simulink model "BuckyWagon_01"  (Simulink 7.5)
settings: Solver=FixedStepDiscrete  StartTime=0.0  StopTime=10.0  RelTol=1e-3
PreLoadFcn:
  | try, eval([bdroot '_setup']); catch, eval('model_setup', ''); end
InitFcn:
  | try, eval([bdroot '_setup']); catch, eval('model_setup', ''); end
undefined symbols (not defined in the file): ECU565, High, Low, miniviewSetup, motohawk_build_version, motohawk_get_faults, motohawk_setup_toolchains, motohawk_trunc_name, motohawk_vardec_config_group, motohawk_vardec_path, tc, True
libraries: MotoHawk_lib x499, simulink x29, motohawk_engine_lib x19, miniview_lib x10, motohawk_control_primitives_lib x8, motohawk_annotations_lib x2
(part 8 of 9)

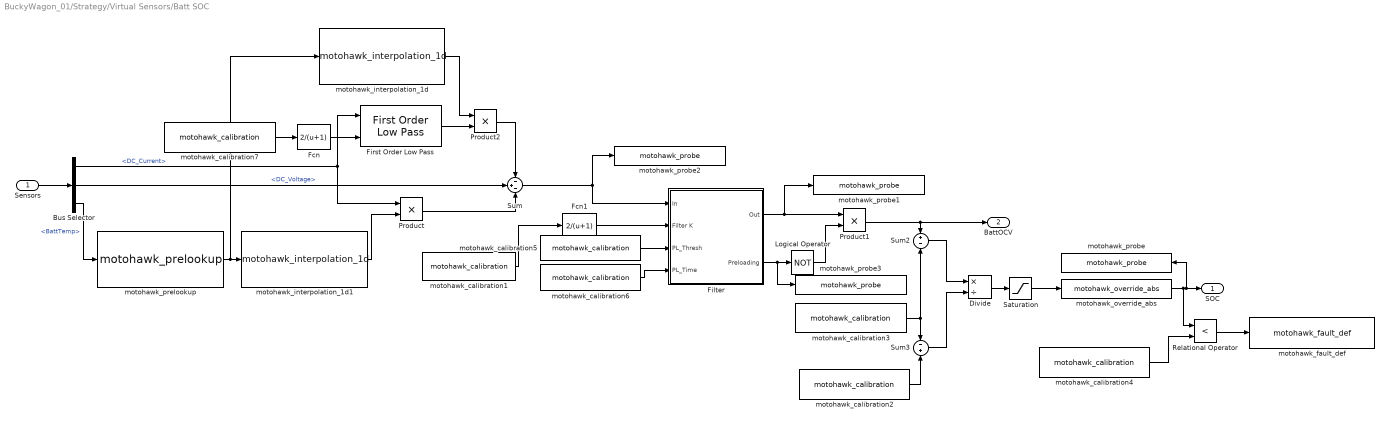
== system BuckyWagon_01/Strategy/Virtual Sensors/Batt SOC ==
  Sensors : Inport  OutDataType=sfix(16)  OutScaling=2^0
  Bus Selector : BusSelector  OutputSignals=DC_Current,DC_Voltage,BattTemp
  Divide : Product  Inputs=*/  OutDataType=sfix(16)  OutScaling=2^-10
  Fcn : Fcn  Expr=2/(u+1)
  Fcn1 : Fcn  Expr=2/(u+1)
  Filter : Subsystem
  First Order Low Pass : motohawk_control_primitives_lib/First Order Low Pass  SystemSampleTime=-1
  Logical Operator : Logic  Operator=NOT  AllPortsSameDT=off  OutDataTypeMode=boolean  OutDataTypeStr=boolean
  Product : Product  OutDataType=sfix(16)  OutScaling=2^0  RndMeth=Zero
  Product1 : Product  OutDataType=sfix(16)  OutScaling=2^0  RndMeth=Zero
  Product2 : Product  OutDataType=sfix(16)  OutScaling=2^0  RndMeth=Zero
  Relational Operator : RelationalOperator  Operator=<  LogicOutDataTypeMode=boolean  OutDataTypeStr=boolean
  Saturation : Saturate  UpperLimit=1  LowerLimit=0  OutDataType=sfix(16)  OutScaling=2^0
  Sum : Sum  Inputs=-+-  OutDataType=sfix(16)  OutScaling=2^0
  Sum2 : Sum  Inputs=+-  OutDataType=sfix(16)  OutScaling=2^0
  Sum3 : Sum  Inputs=-+  OutDataType=sfix(16)  OutScaling=2^0
  motohawk_calibration1 : MotoHawk_lib/Calibration & Probing Blocks/motohawk_calibration  nam='BattV_TC'  val=10/0.005  storage=Calibration  show_more=on  name_source=Use Parameter  data_type=Inherit from 'Default Value'  read_level=1  write_level=1  ovr_cals=on  view_as=Number  enum_struct={'Disabled', 'Enabled'}  vector_style=Wide Row  use_help_units=on  help='Filter on Batt OCV Time Constant.'  units='s'  use_header_enum=off  row_header_enum={}  col_header_enum={}  use_min_max=on  min_val=0.005  max_val=inf  use_precision=on  precision='1.5'  gain=0.005  offset=0  exp=1  use_mototune_group=off  mototune_group=motohawk_vardec_path(gcb)
  motohawk_calibration2 : MotoHawk_lib/Calibration & Probing Blocks/motohawk_calibration  nam='Batt_Full_V'  val=350  storage=Calibration  show_more=on  name_source=Use Parameter  data_type=Inherit from 'Default Value'  read_level=1  write_level=1  ovr_cals=on  view_as=Number  enum_struct={'Disabled', 'Enabled'}  vector_style=Wide Row  use_help_units=on  help='100% SOC Voltage'  units='V'  use_header_enum=off  row_header_enum={}  col_header_enum={}  use_min_max=off  min_val=-inf  max_val=inf  use_precision=on  precision='3.1'  gain=1  offset=0  exp=1  use_mototune_group=off  mototune_group=motohawk_vardec_path(gcb)
  motohawk_calibration3 : MotoHawk_lib/Calibration & Probing Blocks/motohawk_calibration  nam='Batt_Empty_V'  val=350  storage=Calibration  show_more=on  name_source=Use Parameter  data_type=Inherit from 'Default Value'  read_level=1  write_level=1  ovr_cals=on  view_as=Number  enum_struct={'Disabled', 'Enabled'}  vector_style=Wide Row  use_help_units=on  help='0% SOC Voltage'  units='V'  use_header_enum=off  row_header_enum={}  col_header_enum={}  use_min_max=off  min_val=-inf  max_val=inf  use_precision=on  precision='3.1'  gain=1  offset=0  exp=1  use_mototune_group=off  mototune_group=motohawk_vardec_path(gcb)
  motohawk_calibration4 : MotoHawk_lib/Calibration & Probing Blocks/motohawk_calibration  nam='SOC_Dead'  val=0.1  storage=Calibration  show_more=on  name_source=Use Parameter  data_type=Inherit from 'Default Value'  read_level=1  write_level=1  ovr_cals=on  view_as=Number  enum_struct={'Disabled', 'Enabled'}  vector_style=Wide Row  use_help_units=on  help='Below this SOC a Batt Dead fault will occur.'  units='%'  use_header_enum=off  row_header_enum={}  col_header_enum={}  use_min_max=on  min_val=0  max_val=1  use_precision=on  precision='1.3'  gain=1  offset=0  exp=1  use_mototune_group=off  mototune_group=motohawk_vardec_path(gcb)
  motohawk_calibration5 : MotoHawk_lib/Calibration & Probing Blocks/motohawk_calibration  nam='BattVFilt_PreLThres'  val=100  storage=Calibration  show_more=on  name_source=Use Parameter  data_type=Inherit from 'Default Value'  read_level=1  write_level=1  ovr_cals=on  view_as=Number  enum_struct={'Disabled', 'Enabled'}  vector_style=Wide Row  use_help_units=on  help='Below this voltage the filter will preload.'  units='V'  use_header_enum=off  row_header_enum={}  col_header_enum={}  use_min_max=off  min_val=-inf  max_val=inf  use_precision=on  precision=''  gain=1  offset=0  exp=1  use_mototune_group=off  mototune_group=motohawk_vardec_path(gcb)
  motohawk_calibration6 : MotoHawk_lib/Calibration & Probing Blocks/motohawk_calibration  nam='BattVFilt_PreLTime'  val=20  storage=Calibration  show_more=on  name_source=Use Parameter  data_type=Inherit from 'Default Value'  read_level=1  write_level=1  ovr_cals=on  view_as=Number  enum_struct={'Disabled', 'Enabled'}  vector_style=Wide Row  use_help_units=on  help='Filter will preload this long after the threshold is met.'  units='s'  use_header_enum=off  row_header_enum={}  col_header_enum={}  use_min_max=off  min_val=-inf  max_val=inf  use_precision=on  precision='1.3'  gain=0.005  offset=0  exp=1  use_mototune_group=off  mototune_group=motohawk_vardec_path(gcb)
  motohawk_calibration7 : MotoHawk_lib/Calibration & Probing Blocks/motohawk_calibration  nam='Batt_Pol_TC'  val=25/0.005  storage=Calibration  show_more=on  name_source=Use Parameter  data_type=Inherit from 'Default Value'  read_level=1  write_level=1  ovr_cals=on  view_as=Number  enum_struct={'Disabled', 'Enabled'}  vector_style=Wide Row  use_help_units=on  help='Battery Polarization curent TC.'  units='s'  use_header_enum=off  row_header_enum={}  col_header_enum={}  use_min_max=off  min_val=-inf  max_val=inf  use_precision=on  precision='1.3'  gain=0.005  offset=0  exp=1  use_mototune_group=off  mototune_group=motohawk_vardec_path(gcb)
  motohawk_fault_def : MotoHawk_lib/Fault Management Blocks/motohawk_fault_def  nam='BattDead'  mode=Sticky  id=[]  x=5/0.005  y=10/0.005  input_suspected=on  indeterminate=off  increment_xy=on  downsample_count=1  ovr_cals=on  ovr_actions=on  show_actions=off  action1_name=''  action1_cond=(None)  action2_name=''  action2_cond=(None)  action3_name=''  action3_cond=(None)  action4_name=''  action4_cond=(None)
  motohawk_interpolation_1d : MotoHawk_lib/Lookup Tables/motohawk_interpolation_1d  nam='Batt_Pol_Res'  table_data=[0.162 0.1 0.038 0.023]*12/7  show_more=on  data_type=Inherit from 'Table Data'  storage=NonAdaptive  read_level=1  write_level=1  ovr_cals=on  use_help=on  help='Battery internal resistance for polarization resistance.'  units='Ohms'  use_min_max=off  min_val=-inf  max_val=inf  use_precision=on  precision='1.4'  gain=1  offset=0  exp=1  use_links=off  prelookup_block=''  output_name=''  use_mototune_group=off  mototune_group=motohawk_vardec_path(gcb)
  motohawk_interpolation_1d1 : MotoHawk_lib/Lookup Tables/motohawk_interpolation_1d  nam='Batt_Res'  table_data=[0.338 0.2355 0.133 0.108]*12/7  show_more=on  data_type=Inherit from 'Table Data'  storage=NonAdaptive  read_level=1  write_level=1  ovr_cals=on  use_help=on  help='Battery internal resistance.'  units='Ohms'  use_min_max=off  min_val=-inf  max_val=inf  use_precision=on  precision='1.4'  gain=1  offset=0  exp=1  use_links=off  prelookup_block=''  output_name=''  use_mototune_group=off  mototune_group=motohawk_vardec_path(gcb)
  motohawk_override_abs : MotoHawk_lib/Calibration & Probing Blocks/motohawk_override_abs  SystemSampleTime=-1  parent_name='Batt_SOC'  parent_val=0  show_more=off  name_source=Use Parameter  parent_read_level=1  parent_override_level=1  view_as=Number  enum_struct={'Disabled', 'Enabled'}  use_help_units=off  parent_help=''  parent_units=''  use_min_max=off  parent_min=-inf  parent_max=inf  use_precision=off  parent_precision=''  parent_gain=1  parent_offset=0  parent_exp=1  use_mototune_group=off  parent_group=motohawk_vardec_path(gcb)
  motohawk_prelookup : MotoHawk_lib/Lookup Tables/motohawk_prelookup  nam='BattTemp'  breakpoint_data=[-10 7.5 25 50]  show_more=on  data_type=Inherit from 'Table Data'  storage=NonVolatile  read_level=1  write_level=1  ovr_cals=on  use_help=off  help=''  units=''  use_min_max=off  min_val=-inf  max_val=inf  use_precision=off  precision=''  gain=1  offset=0  exp=1  use_links=off  input_name=''  use_mototune_group=off  mototune_group=motohawk_vardec_path(gcb)
  motohawk_probe : MotoHawk_lib/Calibration & Probing Blocks/motohawk_probe  nam='Batt_SOC'  show_more=on  name_source=Use Parameter  read_level=1  view_as=Number  enum_struct={'Disabled', 'Enabled'}  vector_style=Wide Row  use_help_units=off  help=''  units=''  use_header_enum=off  row_header_enum={}  col_header_enum={}  use_precision=on  precision='1.3'  gain=1  offset=0  exp=1  use_mototune_group=off  mototune_group=motohawk_vardec_path(gcb)
  motohawk_probe1 : MotoHawk_lib/Calibration & Probing Blocks/motohawk_probe  nam='Batt_OCV_Filt'  show_more=on  name_source=Use Parameter  read_level=1  view_as=Number  enum_struct={'Disabled', 'Enabled'}  vector_style=Wide Row  use_help_units=off  help=''  units=''  use_header_enum=off  row_header_enum={}  col_header_enum={}  use_precision=on  precision='3.1'  gain=1  offset=0  exp=1  use_mototune_group=off  mototune_group=motohawk_vardec_path(gcb)
  motohawk_probe2 : MotoHawk_lib/Calibration & Probing Blocks/motohawk_probe  nam='Batt_OCV'  show_more=on  name_source=Use Parameter  read_level=1  view_as=Number  enum_struct={'Disabled', 'Enabled'}  vector_style=Wide Row  use_help_units=off  help=''  units=''  use_header_enum=off  row_header_enum={}  col_header_enum={}  use_precision=on  precision='3.1'  gain=1  offset=0  exp=1  use_mototune_group=off  mototune_group=motohawk_vardec_path(gcb)
  motohawk_probe3 : MotoHawk_lib/Calibration & Probing Blocks/motohawk_probe  nam='BattVFilt_PreLoad'  show_more=off  name_source=Use Parameter  read_level=1  view_as=Number  enum_struct={'Disabled', 'Enabled'}  vector_style=Wide Row  use_help_units=off  help=''  units=''  use_header_enum=off  row_header_enum={}  col_header_enum={}  use_precision=off  precision=''  gain=1  offset=0  exp=1  use_mototune_group=off  mototune_group=motohawk_vardec_path(gcb)
  SOC : Outport  OutDataType=sfix(16)  OutScaling=2^0
  BattOCV : Outport  Port=2  OutDataType=sfix(16)  OutScaling=2^0
  wires:
  Sensors/1 -> Bus Selector/1
  motohawk_calibration3/1 -> Sum2/2, Sum3/1
  motohawk_calibration2/1 -> Sum3/2
  Sum2/1 -> Divide/1
  Sum3/1 -> Divide/2
  Divide/1 -> Saturation/1
  motohawk_interpolation_1d1/1 -> Product/2
  motohawk_override_abs/1 -> SOC/1, motohawk_probe/1, Relational Operator/1
  Filter/1(Out) -> motohawk_probe1/1, Product1/1
  Product1/1 -> Sum2/1, BattOCV/1
  Filter/2(Preloading) -> Logical Operator/1, motohawk_probe3/1
  Logical Operator/1 -> Product1/2
  motohawk_calibration5/1 -> Filter/3(PL_Thresh)
  motohawk_calibration6/1 -> Filter/4(PL_Time)
  Bus Selector/1 -> First Order Low Pass/1, Product/1  "<DC_Current>"
  Bus Selector/2 -> Sum/2  "<DC_Voltage>"
  Product/1 -> Sum/3
  First Order Low Pass/1 -> Product2/2
  Product2/1 -> Sum/1
  motohawk_interpolation_1d/1 -> Product2/1
  motohawk_calibration7/1 -> Fcn/1
  Fcn/1 -> First Order Low Pass/2
  Bus Selector/3 -> motohawk_prelookup/1  "<BattTemp>"
  motohawk_prelookup/1 -> motohawk_interpolation_1d1/1, motohawk_interpolation_1d/1
  Sum/1 -> Filter/1(In), motohawk_probe2/1
  Fcn1/1 -> Filter/2(Filter K)
  motohawk_calibration1/1 -> Fcn1/1
  Saturation/1 -> motohawk_override_abs/1
  motohawk_calibration4/1 -> Relational Operator/2
  Relational Operator/1 -> motohawk_fault_def/1

== system BuckyWagon_01/Strategy/Virtual Sensors/Vehicle Speed ==
  Sensors : Inport  OutDataType=sfix(16)  OutScaling=2^0
  Bus Selector : BusSelector  OutputSignals=MotorSpeed
  Product : Product  OutDataType=sfix(16)  OutScaling=2^0  RndMeth=Zero
  motohawk_calibration : MotoHawk_lib/Calibration & Probing Blocks/motohawk_calibration  nam='OveralRatio'  val=1  storage=Calibration  show_more=on  name_source=Use Parameter  data_type=Inherit from 'Default Value'  read_level=1  write_level=1  ovr_cals=on  view_as=Number  enum_struct={'Disabled', 'Enabled'}  vector_style=Wide Row  use_help_units=on  help='Used to calculate vehicle speed from motor speed'  units='mph/rpm'  use_header_enum=off  row_header_enum={}  col_header_enum={}  use_min_max=off  min_val=-inf  max_val=inf  use_precision=on  precision='1.4'  gain=1  offset=0  exp=1  use_mototune_group=off  mototune_group=motohawk_vardec_path(gcb)
  motohawk_override_abs : MotoHawk_lib/Calibration & Probing Blocks/motohawk_override_abs  SystemSampleTime=-1  parent_name='Vehicle_Speed'  parent_val=0  show_more=off  name_source=Use Parameter  parent_read_level=1  parent_override_level=1  view_as=Number  enum_struct={'Disabled', 'Enabled'}  use_help_units=off  parent_help=''  parent_units=''  use_min_max=off  parent_min=-inf  parent_max=inf  use_precision=off  parent_precision=''  parent_gain=1  parent_offset=0  parent_exp=1  use_mototune_group=off  parent_group=motohawk_vardec_path(gcb)
  motohawk_probe : MotoHawk_lib/Calibration & Probing Blocks/motohawk_probe  nam='Vehicle_Speed'  show_more=on  name_source=Use Parameter  read_level=1  view_as=Number  enum_struct={'Disabled', 'Enabled'}  vector_style=Wide Row  use_help_units=off  help=''  units=''  use_header_enum=off  row_header_enum={}  col_header_enum={}  use_precision=on  precision='1.3'  gain=1  offset=0  exp=1  use_mototune_group=off  mototune_group=motohawk_vardec_path(gcb)
  Speed : Outport  OutDataType=sfix(16)  OutScaling=2^0
  wires:
  Sensors/1 -> Bus Selector/1
  Bus Selector/1 -> Product/1  "<MotorSpeed>"
  motohawk_calibration/1 -> Product/2
  Product/1 -> motohawk_override_abs/1
  motohawk_override_abs/1 -> Speed/1, motohawk_probe/1

== system BuckyWagon_01/Main Power Relay/Background/Delay/MotoHawk S-R Flip-Flop ==
  note: MotoHawk S-R Flip-Flop
  S : Inport  OutDataType=sfix(16)  OutScaling=2^0
  R : Inport  Port=2  OutDataType=sfix(16)  OutScaling=2^0
  Logical Operator : Logic  Operator=OR  OutDataTypeMode=boolean  OutDataTypeStr=boolean
  Logical Operator1 : Logic  Operator=NOT  OutDataTypeMode=boolean  OutDataTypeStr=boolean
  Logical Operator2 : Logic  OutDataTypeMode=boolean  OutDataTypeStr=boolean
  Logical Operator3 : Logic  Operator=NOT  OutDataTypeMode=boolean  OutDataTypeStr=boolean
  Signal Specification : SignalSpecification  DataType=boolean  OutDataType=sfix(16)  OutScaling=2^0  OutDataTypeStr=boolean
  Signal Specification1 : SignalSpecification  DataType=boolean  OutDataType=sfix(16)  OutScaling=2^0  OutDataTypeStr=boolean
  Unit Delay : UnitDelay  X0=ic_bool  SampleTime=-1
  Q : Outport  OutDataType=sfix(16)  OutScaling=2^0
  !Q : Outport  Port=2  OutDataType=sfix(16)  OutScaling=2^0
  wires:
  Logical Operator3/1 -> !Q/1
  R/1 -> Signal Specification/1
  S/1 -> Signal Specification1/1
  Signal Specification1/1 -> Logical Operator/2
  Signal Specification/1 -> Logical Operator1/1
  Logical Operator2/1 -> Q/1, Unit Delay/1, Logical Operator3/1
  Unit Delay/1 -> Logical Operator/1
  Logical Operator/1 -> Logical Operator2/1
  Logical Operator1/1 -> Logical Operator2/2

== system BuckyWagon_01/Strategy/Actuators/BattIndicator/Enabled Subsystem ==
  Period (Cnt) : Inport  OutDataType=sfix(16)  OutScaling=2^0
  Enable : EnablePort  StatesWhenEnabling=reset
  Constant : Constant  OutDataTypeMode=int16  OutDataType=sfix(16)  OutScaling=2^0  OutDataTypeStr=int16
  Gain : Gain  Gain=0.5  ParameterDataType=sfix(16)  ParameterScaling=2^0  OutDataType=sfix(16)  OutScaling=2^0  OutDataTypeStr=Inherit: Same as input
  Relational Operator : RelationalOperator  Operator=<=  LogicOutDataTypeMode=boolean  OutDataTypeStr=boolean
  Sum : Sum  Inputs=|+-  OutDataType=sfix(16)  OutScaling=2^0
  Switch : Switch  Criteria=u2 > Threshold
  Unit Delay : UnitDelay  SampleTime=-1
  Out : Outport  OutDataType=sfix(16)  OutScaling=2^0
  wires:
  Relational Operator/1 -> Out/1
  Gain/1 -> Relational Operator/1
  Period (Cnt)/1 -> Gain/1, Switch/3
  Switch/1 -> Sum/1
  Sum/1 -> Relational Operator/2, Unit Delay/1
  Unit Delay/1 -> Switch/1, Switch/2
  Constant/1 -> Sum/2

== system BuckyWagon_01/Strategy/Actuators/BrakeInd/Enabled Subsystem ==
  Period (Cnt) : Inport  OutDataType=sfix(16)  OutScaling=2^0
  Enable : EnablePort  StatesWhenEnabling=reset
  Constant : Constant  OutDataTypeMode=int16  OutDataType=sfix(16)  OutScaling=2^0  OutDataTypeStr=int16
  Gain : Gain  Gain=0.5  ParameterDataType=sfix(16)  ParameterScaling=2^0  OutDataType=sfix(16)  OutScaling=2^0  OutDataTypeStr=Inherit: Same as input
  Relational Operator : RelationalOperator  Operator=<=  LogicOutDataTypeMode=boolean  OutDataTypeStr=boolean
  Sum : Sum  Inputs=|+-  OutDataType=sfix(16)  OutScaling=2^0
  Switch : Switch  Criteria=u2 > Threshold
  Unit Delay : UnitDelay  SampleTime=-1
  Out : Outport  OutDataType=sfix(16)  OutScaling=2^0  InitialOutput=[0]
  wires:
  Relational Operator/1 -> Out/1
  Gain/1 -> Relational Operator/1
  Period (Cnt)/1 -> Gain/1, Switch/3
  Switch/1 -> Sum/1
  Sum/1 -> Relational Operator/2, Unit Delay/1
  Unit Delay/1 -> Switch/1, Switch/2
  Constant/1 -> Sum/2

== system BuckyWagon_01/Strategy/Actuators/CheckEngineInd/Enabled Subsystem ==
  Period (Cnt) : Inport  OutDataType=sfix(16)  OutScaling=2^0
  Enable : EnablePort  StatesWhenEnabling=reset
  Constant : Constant  OutDataTypeMode=int16  OutDataType=sfix(16)  OutScaling=2^0  OutDataTypeStr=int16
  Gain : Gain  Gain=0.5  ParameterDataType=sfix(16)  ParameterScaling=2^0  OutDataType=sfix(16)  OutScaling=2^0  OutDataTypeStr=Inherit: Same as input
  Relational Operator : RelationalOperator  Operator=<=  LogicOutDataTypeMode=boolean  OutDataTypeStr=boolean
  Sum : Sum  Inputs=|+-  OutDataType=sfix(16)  OutScaling=2^0
  Switch : Switch  Criteria=u2 > Threshold
  Unit Delay : UnitDelay  SampleTime=-1
  Out : Outport  OutDataType=sfix(16)  OutScaling=2^0  InitialOutput=[0]
  wires:
  Constant/1 -> Sum/2
  Unit Delay/1 -> Switch/2, Switch/1
  Sum/1 -> Unit Delay/1, Relational Operator/2
  Switch/1 -> Sum/1
  Period (Cnt)/1 -> Switch/3, Gain/1
  Gain/1 -> Relational Operator/1
  Relational Operator/1 -> Out/1

== system BuckyWagon_01/Strategy/Actuators/ReverseInd/Enabled Subsystem ==
  Period (Cnt) : Inport  OutDataType=sfix(16)  OutScaling=2^0
  Enable : EnablePort  StatesWhenEnabling=reset
  Constant : Constant  OutDataTypeMode=int16  OutDataType=sfix(16)  OutScaling=2^0  OutDataTypeStr=int16
  Gain : Gain  Gain=0.5  ParameterDataType=sfix(16)  ParameterScaling=2^0  OutDataType=sfix(16)  OutScaling=2^0  OutDataTypeStr=Inherit: Same as input
  Relational Operator : RelationalOperator  Operator=<=  LogicOutDataTypeMode=boolean  OutDataTypeStr=boolean
  Sum : Sum  Inputs=|+-  OutDataType=sfix(16)  OutScaling=2^0
  Switch : Switch  Criteria=u2 > Threshold
  Unit Delay : UnitDelay  SampleTime=-1
  Out : Outport  OutDataType=sfix(16)  OutScaling=2^0  InitialOutput=[0]
  wires:
  Relational Operator/1 -> Out/1
  Gain/1 -> Relational Operator/1
  Period (Cnt)/1 -> Gain/1, Switch/3
  Switch/1 -> Sum/1
  Sum/1 -> Relational Operator/2, Unit Delay/1
  Unit Delay/1 -> Switch/1, Switch/2
  Constant/1 -> Sum/2

== system BuckyWagon_01/Strategy/Actuators/TempIndicator/Enabled Subsystem ==
  Period (Cnt) : Inport  OutDataType=sfix(16)  OutScaling=2^0
  Enable : EnablePort  StatesWhenEnabling=reset
  Constant : Constant  OutDataTypeMode=int16  OutDataType=sfix(16)  OutScaling=2^0  OutDataTypeStr=int16
  Gain : Gain  Gain=0.5  ParameterDataType=sfix(16)  ParameterScaling=2^0  OutDataType=sfix(16)  OutScaling=2^0  OutDataTypeStr=Inherit: Same as input
  Relational Operator : RelationalOperator  Operator=<=  LogicOutDataTypeMode=boolean  OutDataTypeStr=boolean
  Sum : Sum  Inputs=|+-  OutDataType=sfix(16)  OutScaling=2^0
  Switch : Switch  Criteria=u2 > Threshold
  Unit Delay : UnitDelay  SampleTime=-1
  Out : Outport  OutDataType=sfix(16)  OutScaling=2^0
  wires:
  Constant/1 -> Sum/2
  Unit Delay/1 -> Switch/2, Switch/1
  Sum/1 -> Unit Delay/1, Relational Operator/2
  Switch/1 -> Sum/1
  Period (Cnt)/1 -> Switch/3, Gain/1
  Gain/1 -> Relational Operator/1
  Relational Operator/1 -> Out/1

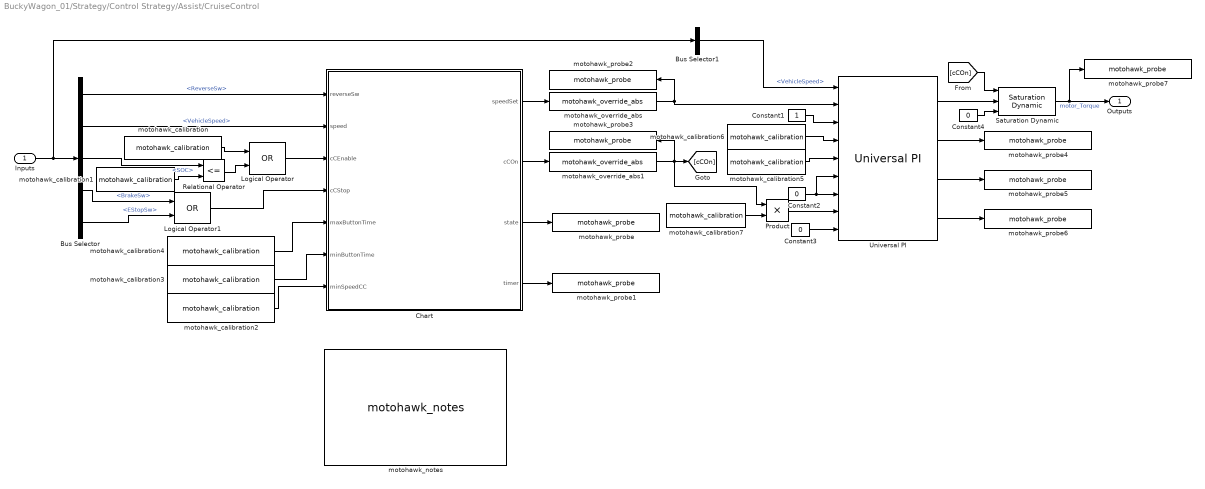
== system BuckyWagon_01/Strategy/Control Strategy/Assist/CruiseControl ==
  Inputs : Inport  OutDataType=sfix(16)  OutScaling=2^0
  Bus Selector : BusSelector  OutputSignals=Physical.ReverseSw,Virtual.VehicleSpeed,Virtual.SOC,Physical.BrakeSw,Physical.EStopSw
  Bus Selector1 : BusSelector  OutputSignals=Virtual.VehicleSpeed
  Chart : Stateflow chart  TreatAsAtomicUnit=on
  Constant1 : Constant  OutDataType=sfix(16)  OutScaling=2^0
  Constant2 : Constant  Value=0  OutDataType=sfix(16)  OutScaling=2^0
  Constant3 : Constant  Value=0  OutDataType=sfix(16)  OutScaling=2^0
  Constant4 : Constant  Value=0  OutDataType=sfix(16)  OutScaling=2^0
  Logical Operator : Logic  Operator=OR  IconShape=distinctive  AllPortsSameDT=off  OutDataTypeMode=boolean  OutDataTypeStr=boolean
  Logical Operator1 : Logic  Operator=OR  IconShape=distinctive  AllPortsSameDT=off  OutDataTypeMode=boolean  OutDataTypeStr=boolean
  Product : Product  OutDataType=sfix(16)  OutScaling=2^0  RndMeth=Zero
  Relational Operator : RelationalOperator  Operator=<=  LogicOutDataTypeMode=boolean  OutDataTypeStr=boolean
  Saturation Dynamic : simulink/Discontinuities/Saturation Dynamic  SystemSampleTime=-1  OutMin=[]  OutMax=[]  OutDataTypeStr=Inherit: Same as second input  OutDataType=sfix(16)  OutScaling=2^-10  DoSatur=off
  Universal PI : motohawk_control_primitives_lib/Universal PI  Description=|  SystemSampleTime=-1  samp_time=-1
      | /* Name: ErrorGain Unit:mult ClassID:VAR StorageID:FLASH Access:RW4+RW3+NA2+NA1 TypeID:UINT4                   
      |    Gain:0.000000001 Min:0.000000000 Max:4.000000000 Format:10.9 UpdateID:REMOTE Help:"This gain is applied to "
      |    "the error term before it is used to calculate the P, I and D terms." VardecSig:6C */                       
      |                                                                                                                
      | /* Name: ITermLowerLim Unit:0 ClassID:VAR StorageID:FLASH Access:RW4+RW3+NA2+NA1 TypeID:SINT2 Gain:0.1         
      |    Min:-3276.8 Max:3276.7 Format:5.1 UpdateID:REMOTE Help:"Lower limit on the I-term value." VardecSig:6C */   
      |                                                                                                                
      | /* Name: ITermUpperLim ClassID:VAR StorageID:FLASH Access:RW4+RW3+NA2+NA1 TypeID:SINT2 Gain:0.1 Min:-3276.8    
      |    Max:3276.7 Format:5.1 UpdateID:REMOTE Help:"Upper limit on I-term value." VardecSig:6C */                   
      |                                                                                                                
      | /* Name: PIDOutLowerLim ClassID:VAR StorageID:FLASH Access:RW4+RW3+NA2+NA1 TypeID:SINT2 Gain:0.1               
      |    Min:-3276.8 Max:3276.7 Format:5.1 UpdateID:REMOTE Help:"Lower limit on PID output." VardecSig:6C */         
      |                                                                                                                
      | /* Name: PIDOutUpperLim ClassID:VAR StorageID:FLASH Access:RW4+RW3+NA2+NA1 TypeID:SINT2 Gain:0.1               
      |    Min:-3276.8 Max:3276.7 Format:3.1 UpdateID:REMOTE Help:"Upper limit on PID output." VardecSig:6C */
  motohawk_calibration : MotoHawk_lib/Calibration & Probing Blocks/motohawk_calibration  nam='cCEnable'  val=0  storage=Calibration  show_more=on  name_source=Use Parameter  data_type=uint8  read_level=1  write_level=1  ovr_cals=on  view_as=Enumeration  enum_struct={'Disabled', 'Enabled'}  vector_style=Wide Row  use_help_units=on  help='Enable Cruise Control.'  units=''  use_header_enum=off  row_header_enum={}  col_header_enum={}  use_min_max=off  min_val=-inf  max_val=inf  use_precision=off  precision=''  gain=1  offset=0  exp=1  use_mototune_group=off  mototune_group=motohawk_vardec_path(gcb)
  motohawk_calibration1 : MotoHawk_lib/Calibration & Probing Blocks/motohawk_calibration  nam='cCMinSOC'  val=0.2  storage=Calibration  show_more=on  name_source=Use Parameter  data_type=Inherit from 'Default Value'  read_level=1  write_level=1  ovr_cals=on  view_as=Number  enum_struct={'Disabled', 'Enabled'}  vector_style=Wide Row  use_help_units=on  help='Minimum SOC for cruise control to work.'  units='%'  use_header_enum=off  row_header_enum={}  col_header_enum={}  use_min_max=on  min_val=0  max_val=1  use_precision=on  precision='1.2'  gain=1  offset=0  exp=1  use_mototune_group=off  mototune_group=motohawk_vardec_path(gcb)
  motohawk_calibration2 : MotoHawk_lib/Calibration & Probing Blocks/motohawk_calibration  nam='cCMinSpeed'  val=20  storage=Calibration  show_more=on  name_source=Use Parameter  data_type=Inherit from 'Default Value'  read_level=1  write_level=1  ovr_cals=on  view_as=Number  enum_struct={'Disabled', 'Enabled'}  vector_style=Wide Row  use_help_units=on  help='Minimum speed for cruise control to work.'  units='mph'  use_header_enum=off  row_header_enum={}  col_header_enum={}  use_min_max=on  min_val=0  max_val=100  use_precision=on  precision='2.1'  gain=1  offset=0  exp=1  use_mototune_group=off  mototune_group=motohawk_vardec_path(gcb)
  motohawk_calibration3 : MotoHawk_lib/Calibration & Probing Blocks/motohawk_calibration  nam='cCMinButtonTime'  val=0.1/0.005  storage=Calibration  show_more=on  name_source=Use Parameter  data_type=uint8  read_level=1  write_level=1  ovr_cals=on  view_as=Number  enum_struct={'Disabled', 'Enabled'}  vector_style=Wide Row  use_help_units=on  help='Minimum time for button press or unpress.'  units='s'  use_header_enum=off  row_header_enum={}  col_header_enum={}  use_min_max=on  min_val=0  max_val=255/0.005  use_precision=on  precision='1.3'  gain=0.005  offset=0  exp=1  use_mototune_group=off  mototune_group=motohawk_vardec_path(gcb)
  motohawk_calibration4 : MotoHawk_lib/Calibration & Probing Blocks/motohawk_calibration  nam='cCMaxButtonTime'  val=0.2/0.005  storage=Calibration  show_more=on  name_source=Use Parameter  data_type=uint8  read_level=1  write_level=1  ovr_cals=on  view_as=Number  enum_struct={'Disabled', 'Enabled'}  vector_style=Wide Row  use_help_units=on  help='Maximum time for button press or unpress.'  units='s'  use_header_enum=off  row_header_enum={}  col_header_enum={}  use_min_max=on  min_val=0  max_val=255/0.005  use_precision=on  precision='1.3'  gain=0.005  offset=0  exp=1  use_mototune_group=off  mototune_group=motohawk_vardec_path(gcb)
  motohawk_calibration5 : MotoHawk_lib/Calibration & Probing Blocks/motohawk_calibration  nam='cCk_I'  val=0  storage=Calibration  show_more=on  name_source=Use Parameter  data_type=Inherit from 'Default Value'  read_level=1  write_level=1  ovr_cals=on  view_as=Number  enum_struct={'Disabled', 'Enabled'}  vector_style=Wide Row  use_help_units=on  help='Integrator gain for cruise control PI.'  units=''  use_header_enum=off  row_header_enum={}  col_header_enum={}  use_min_max=on  min_val=0  max_val=1  use_precision=on  precision='1.4'  gain=1  offset=0  exp=1  use_mototune_group=off  mototune_group=motohawk_vardec_path(gcb)
  motohawk_calibration6 : MotoHawk_lib/Calibration & Probing Blocks/motohawk_calibration  nam='cCk_P'  val=0  storage=Calibration  show_more=on  name_source=Use Parameter  data_type=Inherit from 'Default Value'  read_level=1  write_level=1  ovr_cals=on  view_as=Number  enum_struct={'Disabled', 'Enabled'}  vector_style=Wide Row  use_help_units=on  help='Integrator gain for cruise control PI.'  units=''  use_header_enum=off  row_header_enum={}  col_header_enum={}  use_min_max=on  min_val=0  max_val=1  use_precision=on  precision='1.4'  gain=1  offset=0  exp=1  use_mototune_group=off  mototune_group=motohawk_vardec_path(gcb)
  motohawk_calibration7 : MotoHawk_lib/Calibration & Probing Blocks/motohawk_calibration  nam='cCk_MaxAccel'  val=0  storage=Calibration  show_more=on  name_source=Use Parameter  data_type=Inherit from 'Default Value'  read_level=1  write_level=1  ovr_cals=on  view_as=Number  enum_struct={'Disabled', 'Enabled'}  vector_style=Wide Row  use_help_units=on  help='Maximum Torque the cruise control can request.'  units='%'  use_header_enum=off  row_header_enum={}  col_header_enum={}  use_min_max=on  min_val=0  max_val=1  use_precision=on  precision='1.3'  gain=1  offset=0  exp=1  use_mototune_group=off  mototune_group=motohawk_vardec_path(gcb)
  motohawk_notes : motohawk_annotations_lib/motohawk_notes  BlockType_='Mototron_Notes'  desc=' \newline\fontsize{18}\bfCruise Control State\rm\fontsize{12}\newline\newline0 - Disabled\newline1 - Off\newline2 - PressOne\newline3 - WaitOne\newline4 - PressTwo\newline5 - On'  edit_text=' \newline\fontsize{18}\bfCruise Control State\rm\fontsize{12}\newline\newline0 - Disabled\newline1 - Off\newline2 - PressOne\newline3 - WaitOne\newline4 - PressTwo\newline5 - On'  edit_as=6
  motohawk_override_abs : MotoHawk_lib/Calibration & Probing Blocks/motohawk_override_abs  SystemSampleTime=-1  parent_name='cCSpeedSet'  parent_val=0  show_more=on  name_source=Use Parameter  parent_read_level=1  parent_override_level=1  view_as=Number  enum_struct={'Disabled', 'Enabled'}  use_help_units=off  parent_help=''  parent_units=''  use_min_max=off  parent_min=-inf  parent_max=inf  use_precision=on  parent_precision='1.1'  parent_gain=1  parent_offset=0  parent_exp=1  use_mototune_group=off  parent_group=motohawk_vardec_path(gcb)
  motohawk_override_abs1 : MotoHawk_lib/Calibration & Probing Blocks/motohawk_override_abs  SystemSampleTime=-1  parent_name='cCOn'  parent_val=0  show_more=on  name_source=Use Parameter  parent_read_level=1  parent_override_level=1  view_as=Number  enum_struct={'Disabled', 'Enabled'}  use_help_units=off  parent_help=''  parent_units=''  use_min_max=off  parent_min=-inf  parent_max=inf  use_precision=on  parent_precision='1.0'  parent_gain=1  parent_offset=0  parent_exp=1  use_mototune_group=off  parent_group=motohawk_vardec_path(gcb)
  motohawk_probe : MotoHawk_lib/Calibration & Probing Blocks/motohawk_probe  nam='cCState'  show_more=on  name_source=Use Parameter  read_level=1  view_as=Enumeration  enum_struct={'Disabled','Off','Press1','Wait1','Press2','On'}  vector_style=Wide Row  use_help_units=off  help=''  units=''  use_header_enum=off  row_header_enum={}  col_header_enum={}  use_precision=off  precision=''  gain=1  offset=0  exp=1  use_mototune_group=off  mototune_group=motohawk_vardec_path(gcb)
  motohawk_probe1 : MotoHawk_lib/Calibration & Probing Blocks/motohawk_probe  nam='cCTimer'  show_more=on  name_source=Use Parameter  read_level=1  view_as=Number  enum_struct={'Disabled','Off','Press1','Wait1','Press2','On'}  vector_style=Wide Row  use_help_units=off  help=''  units=''  use_header_enum=off  row_header_enum={}  col_header_enum={}  use_precision=on  precision='1.3'  gain=0.005  offset=0  exp=1  use_mototune_group=off  mototune_group=motohawk_vardec_path(gcb)
  motohawk_probe2 : MotoHawk_lib/Calibration & Probing Blocks/motohawk_probe  nam='cCSpeedSet'  show_more=on  name_source=Use Parameter  read_level=1  view_as=Number  enum_struct={'Disabled','Off','Press1','Wait1','Press2','On'}  vector_style=Wide Row  use_help_units=off  help=''  units=''  use_header_enum=off  row_header_enum={}  col_header_enum={}  use_precision=on  precision='1.1'  gain=1  offset=0  exp=1  use_mototune_group=off  mototune_group=motohawk_vardec_path(gcb)
  motohawk_probe3 : MotoHawk_lib/Calibration & Probing Blocks/motohawk_probe  nam='cCOn'  show_more=on  name_source=Use Parameter  read_level=1  view_as=Number  enum_struct={'Disabled','Off','Press1','Wait1','Press2','On'}  vector_style=Wide Row  use_help_units=off  help=''  units=''  use_header_enum=off  row_header_enum={}  col_header_enum={}  use_precision=on  precision='1.0'  gain=1  offset=0  exp=1  use_mototune_group=off  mototune_group=motohawk_vardec_path(gcb)
  motohawk_probe4 : MotoHawk_lib/Calibration & Probing Blocks/motohawk_probe  nam='cCError'  show_more=on  name_source=Use Parameter  read_level=1  view_as=Number  enum_struct={'Disabled','Off','Press1','Wait1','Press2','On'}  vector_style=Wide Row  use_help_units=off  help=''  units=''  use_header_enum=off  row_header_enum={}  col_header_enum={}  use_precision=on  precision='1.3'  gain=1  offset=0  exp=1  use_mototune_group=off  mototune_group=motohawk_vardec_path(gcb)
  motohawk_probe5 : MotoHawk_lib/Calibration & Probing Blocks/motohawk_probe  nam='cCP_Term'  show_more=on  name_source=Use Parameter  read_level=1  view_as=Number  enum_struct={'Disabled','Off','Press1','Wait1','Press2','On'}  vector_style=Wide Row  use_help_units=off  help=''  units=''  use_header_enum=off  row_header_enum={}  col_header_enum={}  use_precision=on  precision='1.3'  gain=1  offset=0  exp=1  use_mototune_group=off  mototune_group=motohawk_vardec_path(gcb)
  motohawk_probe6 : MotoHawk_lib/Calibration & Probing Blocks/motohawk_probe  nam='cCI_Term'  show_more=on  name_source=Use Parameter  read_level=1  view_as=Number  enum_struct={'Disabled','Off','Press1','Wait1','Press2','On'}  vector_style=Wide Row  use_help_units=off  help=''  units=''  use_header_enum=off  row_header_enum={}  col_header_enum={}  use_precision=on  precision='1.3'  gain=1  offset=0  exp=1  use_mototune_group=off  mototune_group=motohawk_vardec_path(gcb)
  motohawk_probe7 : MotoHawk_lib/Calibration & Probing Blocks/motohawk_probe  nam='cCTrqReq'  show_more=on  name_source=Use Parameter  read_level=1  view_as=Number  enum_struct={'Disabled','Off','Press1','Wait1','Press2','On'}  vector_style=Wide Row  use_help_units=off  help=''  units=''  use_header_enum=off  row_header_enum={}  col_header_enum={}  use_precision=on  precision='1.3'  gain=1  offset=0  exp=1  use_mototune_group=off  mototune_group=motohawk_vardec_path(gcb)
  Outputs : Outport  OutDataType=sfix(16)  OutScaling=2^0
  wires:
  Saturation Dynamic/1 -> Outputs/1, motohawk_probe7/1  "motor_Torque"
  Inputs/1 -> Bus Selector/1, Bus Selector1/1
  Bus Selector/1 -> Chart/1(reverseSw)  "<ReverseSw>"
  Bus Selector/2 -> Chart/2(speed)  "<VehicleSpeed>"
  motohawk_calibration1/1 -> Relational Operator/2
  motohawk_calibration2/1 -> Chart/7(minSpeedCC)
  Logical Operator/1 -> Chart/3(cCEnable)
  motohawk_calibration/1 -> Logical Operator/1
  Relational Operator/1 -> Logical Operator/2
  Bus Selector/3 -> Relational Operator/1  "<SOC>"
  Bus Selector/4 -> Logical Operator1/1  "<BrakeSw>"
  Bus Selector/5 -> Logical Operator1/2  "<EStopSw>"
  Logical Operator1/1 -> Chart/4(cCStop)
  motohawk_calibration4/1 -> Chart/5(maxButtonTime)
  motohawk_calibration3/1 -> Chart/6(minButtonTime)
  Chart/3(state) -> motohawk_probe/1
  Chart/4(timer) -> motohawk_probe1/1
  Chart/1(speedSet) -> motohawk_override_abs/1
  motohawk_override_abs/1 -> motohawk_probe2/1, Universal PI/2
  Chart/2(cCOn) -> motohawk_override_abs1/1
  motohawk_override_abs1/1 -> motohawk_probe3/1, Product/1, [cCOn]
  motohawk_calibration5/1 -> Universal PI/5
  motohawk_calibration6/1 -> Universal PI/4
  Constant1/1 -> Universal PI/3
  Constant2/1 -> Universal PI/6, Universal PI/7
  Constant3/1 -> Universal PI/9
  Product/1 -> Universal PI/8
  motohawk_calibration7/1 -> Product/2
  Universal PI/1 -> Saturation Dynamic/2
  Universal PI/2 -> motohawk_probe4/1
  Universal PI/3 -> motohawk_probe5/1
  Universal PI/4 -> motohawk_probe6/1
  Bus Selector1/1 -> Universal PI/1  "<VehicleSpeed>"
  Constant4/1 -> Saturation Dynamic/3
  [cCOn] -> Saturation Dynamic/1

== system BuckyWagon_01/Strategy/Control Strategy/Assist/StallTorqueFault ==
  Inputs : Inport  OutDataType=sfix(16)  OutScaling=2^0
  Torque : Inport  Port=2  OutDataType=sfix(16)  OutScaling=2^0
  Abs : Abs  OutDataType=sfix(16)  OutScaling=2^0
  Bus Selector : BusSelector  OutputSignals=Physical.Accel,Virtual.VehicleSpeed
  Constant : Constant  OutDataType=sfix(16)  OutScaling=2^0
  Constant1 : Constant  Value=-1  OutDataType=sfix(16)  OutScaling=2^0
  Constant2 : Constant  Value=0  OutDataType=sfix(16)  OutScaling=2^0
  Constant3 : Constant  Value=0  OutDataType=sfix(16)  OutScaling=2^0
  Constant4 : Constant  Value=0  OutDataType=sfix(16)  OutScaling=2^0
  Hysterisis : Subsystem  AncestorBlock=motohawk_control_primitives_lib/Hysterisis
      mask Display:
      | patch([0 0 1 1], [0 0.075 0.075 0], [230/255 0/255 0/255])
      | patch([0 0 1 1], [0.025 0.05 0.05 0.025], [150/255 0/255 0/255])
      | patch([0 0 1 1], [0 0.025 0.025 0], [0/255 0/255 0/255])
      | 
      | disp('HYSTERISIS')
  Integrator : motohawk_control_primitives_lib/Integrator  SystemSampleTime=-1  samp_time=0.005
  Product : Product  OutDataType=sfix(16)  OutScaling=2^0  RndMeth=Zero
  Relational Operator : RelationalOperator  Operator=<=  LogicOutDataTypeMode=boolean  OutDataTypeStr=boolean
  Relational Operator2 : RelationalOperator  Operator=>  LogicOutDataTypeMode=boolean  OutDataTypeStr=boolean
  Sum : Sum  Inputs=-+|  OutDataType=sfix(16)  OutScaling=2^0
  Switch : Switch  Criteria=u2 ~= 0  OutDataType=sfix(16)  OutScaling=2^0
  Switch1 : Switch  Criteria=u2 ~= 0  OutDataType=sfix(16)  OutScaling=2^0
  motohawk_calibration : MotoHawk_lib/Calibration & Probing Blocks/motohawk_calibration  nam='StallSpd'  val=1  storage=Calibration  show_more=on  name_source=Use Parameter  data_type=Inherit from 'Default Value'  read_level=1  write_level=1  ovr_cals=on  view_as=Number  enum_struct={'Disabled', 'Enabled'}  vector_style=Wide Row  use_help_units=on  help='Below this vehicle speed is concidered locked rotor.'  units='mph'  use_header_enum=off  row_header_enum={}  col_header_enum={}  use_min_max=on  min_val=0  max_val=100  use_precision=off  precision=''  gain=1  offset=0  exp=1  use_mototune_group=off  mototune_group=motohawk_vardec_path(gcb)
  motohawk_calibration1 : MotoHawk_lib/Calibration & Probing Blocks/motohawk_calibration  nam='StallTrqThres'  val=5  storage=Calibration  show_more=on  name_source=Use Parameter  data_type=Inherit from 'Default Value'  read_level=1  write_level=1  ovr_cals=on  view_as=Number  enum_struct={'Disabled', 'Enabled'}  vector_style=Wide Row  use_help_units=on  help='% seconds of torque allowed while speed is below thres.'  units='% s'  use_header_enum=off  row_header_enum={}  col_header_enum={}  use_min_max=off  min_val=-inf  max_val=inf  use_precision=off  precision=''  gain=1  offset=0  exp=1  use_mototune_group=off  mototune_group=motohawk_vardec_path(gcb)
  motohawk_calibration2 : MotoHawk_lib/Calibration & Probing Blocks/motohawk_calibration  nam='AccelRstThres'  val=0.05  storage=Calibration  show_more=on  name_source=Use Parameter  data_type=Inherit from 'Default Value'  read_level=1  write_level=1  ovr_cals=on  view_as=Number  enum_struct={'Disabled', 'Enabled'}  vector_style=Wide Row  use_help_units=on  help='Below this accel position fault can reset.'  units='%'  use_header_enum=off  row_header_enum={}  col_header_enum={}  use_min_max=on  min_val=0  max_val=1  use_precision=on  precision='1.2'  gain=1  offset=0  exp=1  use_mototune_group=off  mototune_group=motohawk_vardec_path(gcb)
  motohawk_calibration3 : MotoHawk_lib/Calibration & Probing Blocks/motohawk_calibration  nam='AccelRstSpd'  val=2  storage=Calibration  show_more=on  name_source=Use Parameter  data_type=Inherit from 'Default Value'  read_level=1  write_level=1  ovr_cals=on  view_as=Number  enum_struct={'Disabled', 'Enabled'}  vector_style=Wide Row  use_help_units=on  help='%'  units='Rate at which fault is cleared when accel is below thres.'  use_header_enum=off  row_header_enum={}  col_header_enum={}  use_min_max=off  min_val=-inf  max_val=inf  use_precision=off  precision=''  gain=1  offset=0  exp=1  use_mototune_group=off  mototune_group=motohawk_vardec_path(gcb)
  motohawk_fault_def : MotoHawk_lib/Fault Management Blocks/motohawk_fault_def  nam='LockedRotor'  mode=Enabled  id=[]  x=25  y=50  input_suspected=on  indeterminate=off  increment_xy=on  downsample_count=1  ovr_cals=on  ovr_actions=on  show_actions=on  action1_name='DisableDrive'  action1_cond=Suspected or Active  action2_name=''  action2_cond=(None)  action3_name=''  action3_cond=(None)  action4_name=''  action4_cond=(None)
  motohawk_probe : MotoHawk_lib/Calibration & Probing Blocks/motohawk_probe  nam='IntStallTorque'  show_more=off  name_source=Use Parameter  read_level=1  view_as=Number  enum_struct={'Disabled', 'Enabled'}  vector_style=Wide Row  use_help_units=off  help=''  units=''  use_header_enum=off  row_header_enum={}  col_header_enum={}  use_precision=off  precision=''  gain=1  offset=0  exp=1  use_mototune_group=off  mototune_group=motohawk_vardec_path(gcb)
  wires:
  Inputs/1 -> Bus Selector/1
  Bus Selector/2 -> Abs/1  "<VehicleSpeed>"
  motohawk_calibration/1 -> Relational Operator/2
  Relational Operator/1 -> Switch/2
  Switch/1 -> Product/1
  Torque/1 -> Product/2
  Integrator/1 -> Hysterisis/3(Signal), motohawk_probe/1
  motohawk_calibration1/1 -> Integrator/5, Hysterisis/1(HiThresh)
  Constant/1 -> Switch/1
  Constant1/1 -> Switch/3
  motohawk_calibration2/1 -> Relational Operator2/1
  Bus Selector/1 -> Relational Operator2/2  "<Accel>"
  Relational Operator2/1 -> Switch1/2
  motohawk_calibration3/1 -> Switch1/1
  Constant2/1 -> Switch1/3
  Switch1/1 -> Sum/1
  Product/1 -> Sum/2
  Sum/1 -> Integrator/1
  Constant3/1 -> Integrator/2, Integrator/3, Integrator/4
  Constant4/1 -> Hysterisis/2(LowThresh)
  Hysterisis/1(Threshold) -> motohawk_fault_def/1
  Abs/1 -> Relational Operator/1

== system BuckyWagon_01/Strategy/Control Strategy/Contacter Controller/Delay ==
  note: Delay the rising and falling of a boolean signal
  In : Inport  OutDataType=sfix(16)  OutScaling=2^0
  Constant1 : Constant  Value=0  OutDataType=sfix(16)  OutScaling=2^0  OutDataTypeStr=Inherit: Inherit via back propagation
  Constant3 : Constant  Value=0  OutDataType=sfix(16)  OutScaling=2^0  OutDataTypeStr=Inherit: Inherit via back propagation
  Data Type Conversion : DataTypeConversion  OutDataType=sfix(16)  OutScaling=2^0  RndMeth=Zero
  Data Type Conversion1 : DataTypeConversion  OutDataType=sfix(16)  OutScaling=2^0  RndMeth=Zero
  Logical Operator : Logic  Operator=NOT  OutDataTypeMode=boolean  OutDataTypeStr=boolean
  Logical Operator1 : Logic  OutDataTypeMode=boolean  OutDataTypeStr=boolean
  Logical Operator2 : Logic  OutDataTypeMode=boolean  OutDataTypeStr=boolean
  MotoHawk S-R Flip-Flop : Subsystem  mask(MotoHawk S-R Flip-Flop){ic_bool=false}
      mask prompts: ic_bool "Initial condition Q (boolean)"
      mask help:
      | When input S (set) is TRUE, output Q is TRUE (and latched until reset).
      | When input R (reset) is TRUE, output Q is FALSE (and latched until set).
      | If both inputs S and R are TRUE, output Q is FALSE (reset wins).
      mask Display:
      | patch([0 0 1 1], [0 0.075 0.075 0], [230/255 0/255 0/255])
      | patch([0 0 1 1], [0.025 0.05 0.05 0.025], [150/255 0/255 0/255])
      | patch([0 0 1 1], [0 0.025 0.025 0], [0/255 0/255 0/255])
  Relational Operator1 : RelationalOperator  LogicOutDataTypeMode=boolean  OutDataTypeStr=boolean  ZeroCross=off  InputSameDT=on
  Relational Operator2 : RelationalOperator  LogicOutDataTypeMode=boolean  OutDataTypeStr=boolean  ZeroCross=off  InputSameDT=on
  Sum : Sum  Inputs=++|  OutDataType=sfix(16)  OutScaling=2^0  RndMeth=Zero  SaturateOnIntegerOverflow=on  InputSameDT=on
  Sum1 : Sum  Inputs=++|  OutDataType=sfix(16)  OutScaling=2^0  RndMeth=Zero  SaturateOnIntegerOverflow=on  InputSameDT=on
  Switch : Switch  Criteria=u2 ~= 0  Threshold=1  RndMeth=Zero  ZeroCross=off  InputSameDT=on
  Switch1 : Switch  Criteria=u2 ~= 0  Threshold=1  RndMeth=Zero  ZeroCross=off  InputSameDT=on
  Terminator : Terminator
  Unit Delay : UnitDelay  SampleTime=-1
  Unit Delay1 : UnitDelay  SampleTime=-1
  off delay : Constant  Value=10  OutDataType=sfix(16)  OutScaling=2^0
  on delay : Constant  Value=0  OutDataType=sfix(16)  OutScaling=2^0
  Out : Outport  OutDataType=sfix(16)  OutScaling=2^0
  wires:
  Logical Operator1/1 -> MotoHawk S-R Flip-Flop/2(R)
  Logical Operator2/1 -> MotoHawk S-R Flip-Flop/1(S)
  Relational Operator1/1 -> Logical Operator2/2
  Relational Operator2/1 -> Logical Operator1/2
  MotoHawk S-R Flip-Flop/2(!Q) -> Terminator/1
  MotoHawk S-R Flip-Flop/1(Q) -> Out/1
  off delay/1 -> Relational Operator2/2
  Logical Operator/1 -> Logical Operator1/1, Switch1/2, Data Type Conversion1/1
  Data Type Conversion1/1 -> Sum1/2  "0 to 1"
  Sum1/1 -> Switch1/1  "0 to 65535 (saturate hi)"
  Constant3/1 -> Switch1/3
  Switch1/1 -> Relational Operator2/1, Unit Delay1/1  "0 to 65535"
  In/1 -> Logical Operator/1, Logical Operator2/1, Switch/2, Data Type Conversion/1
  Data Type Conversion/1 -> Sum/2  "0 to 1"
  Sum/1 -> Switch/1  "0 to 65535 (saturate hi)"
  Constant1/1 -> Switch/3
  Switch/1 -> Unit Delay/1, Relational Operator1/1  "0 to 65535"
  on delay/1 -> Relational Operator1/2
  Unit Delay1/1 -> Sum1/1  "0 to 65535"
  Unit Delay/1 -> Sum/1  "0 to 65535"

== system BuckyWagon_01/Strategy/Control Strategy/Regen/SOC_RampOut ==
  Torque_In : Inport  OutDataType=sfix(16)  OutScaling=2^0
  SOC : Inport  Port=2  OutDataType=sfix(16)  OutScaling=2^0
  Constant : Constant  OutDataType=sfix(16)  OutScaling=2^0
  Divide : Product  Inputs=*/  OutDataType=sfix(16)  OutScaling=2^-10
  Product : Product  OutDataType=sfix(16)  OutScaling=2^0  RndMeth=Zero
  Relational Operator : RelationalOperator  Operator=<=  LogicOutDataTypeMode=boolean  OutDataTypeStr=boolean
  Saturation : Saturate  UpperLimit=1  LowerLimit=0
  Sum : Sum  Inputs=-++  OutDataType=sfix(16)  OutScaling=2^0
  Switch : Switch  Criteria=u2 ~= 0
  motohawk_calibration : MotoHawk_lib/Calibration & Probing Blocks/motohawk_calibration  nam='RegenSOCRampWidth'  val=0.1  storage=Calibration  show_more=on  name_source=Use Parameter  data_type=Inherit from 'Default Value'  read_level=1  write_level=1  ovr_cals=on  view_as=Number  enum_struct={'Disabled', 'Enabled'}  vector_style=Wide Row  use_help_units=on  help='Regen ramps out this fast over max SOC'  units='%'  use_header_enum=off  row_header_enum={}  col_header_enum={}  use_min_max=on  min_val=0  max_val=1  use_precision=on  precision='1.3'  gain=1  offset=0  exp=1  use_mototune_group=off  mototune_group=motohawk_vardec_path(gcb)
  motohawk_calibration1 : MotoHawk_lib/Calibration & Probing Blocks/motohawk_calibration  nam='RegenMaxSOC'  val=0.10  storage=Calibration  show_more=on  name_source=Use Parameter  data_type=Inherit from 'Default Value'  read_level=1  write_level=1  ovr_cals=on  view_as=Number  enum_struct={'Disabled', 'Enabled'}  vector_style=Wide Row  use_help_units=on  help='Max SOC to Regen At'  units='%'  use_header_enum=off  row_header_enum={}  col_header_enum={}  use_min_max=off  min_val=0  max_val=1  use_precision=on  precision='1.2'  gain=1  offset=0  exp=1  use_mototune_group=off  mototune_group=motohawk_vardec_path(gcb)
  Torque_Out : Outport  OutDataType=sfix(16)  OutScaling=2^0
  wires:
  Saturation/1 -> Product/2
  motohawk_calibration1/1 -> Relational Operator/2, Sum/2
  SOC/1 -> Relational Operator/1, Sum/1
  Sum/1 -> Divide/1
  motohawk_calibration/1 -> Sum/3, Divide/2
  Relational Operator/1 -> Switch/2
  Divide/1 -> Switch/3
  Constant/1 -> Switch/1
  Torque_In/1 -> Product/1
  Switch/1 -> Saturation/1
  Product/1 -> Torque_Out/1
